simulink model "FIXEDPOINT_SECOND_ORDER_SIGMADELTA_QUANTIZED"  (R2021b)
settings: Solver=VariableStepAuto  StartTime=0.0  StopTime=0.01  MaxStep=1e-8  RelTol=1e-3
libraries: fl_lib x9, nesl_utility x4, dspmlti4 x1
settings Model: FPTShortcutValueString='{{},{''BaselineRun'',1,1,1,''BaselineRun'','''',{},''M'','''',''''},{''EmbeddedRun'',1,1,1,''EmbeddedRun'','''',{},''M'','''',''''}}'  Creator=caccolillo  LastModifiedBy=caccolillo
settings OptimizationCC: BlockReduction=off  ConditionallyExecuteInputs=off
settings DebuggingCC: SignalRangeChecking=warning

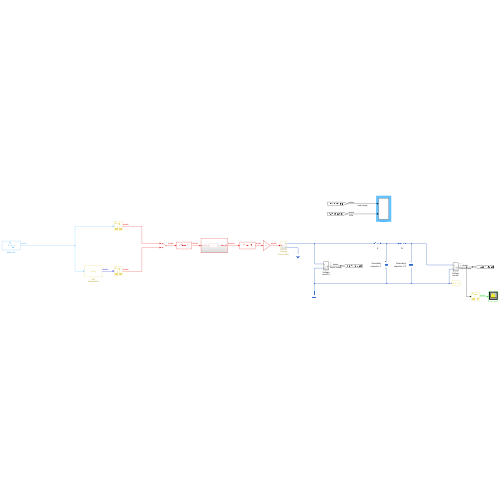
[thumbnail: Simulink's stored preview of the top-level diagram]
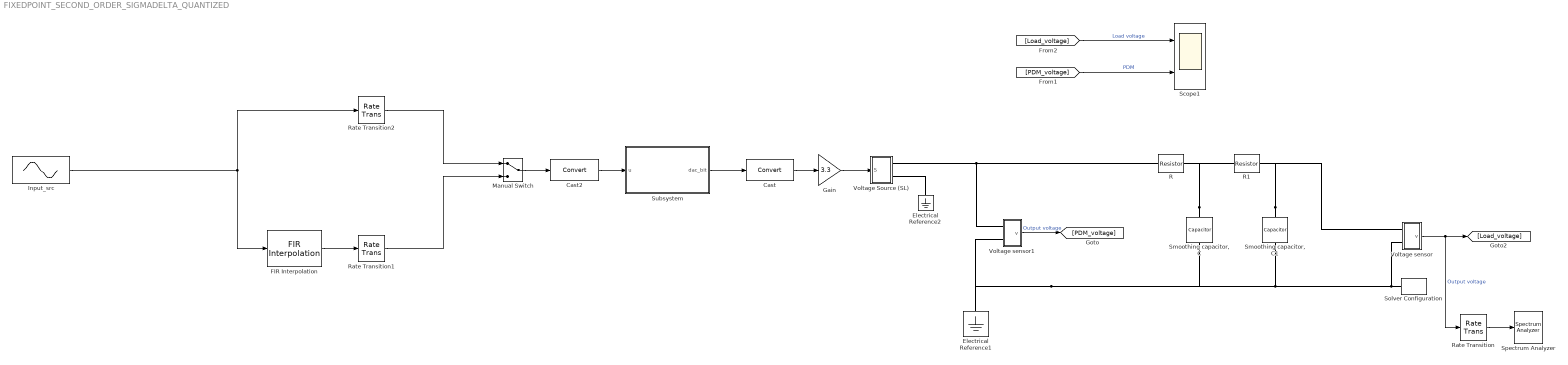
== system FIXEDPOINT_SECOND_ORDER_SIGMADELTA_QUANTIZED ==
  Cast : DataTypeConversion
  Cast2 : DataTypeConversion
  Electrical Reference1 : fl_lib/Electrical/Electrical Elements/Electrical Reference
  Electrical Reference2 : fl_lib/Electrical/Electrical Elements/Electrical Reference
  FIR Interpolation : dspmlti4/FIR Interpolation  FilterSource=Dialog parameters  PrivateCoeffs=0  h=[0.25 0.5 0.75 1.0 0.75 0.5 0.25]  L=4  FilterObject=FINTERP  framing=Allow multirate processing  outputBufInitCond=0  roundingMode=Floor  overflowMode=off  firstCoeffDataTypeStr=Inherit: Same word length as input  firstCoeffMin=[]  firstCoeffMax=[]  firstCoeffLastDataTypeStr=Inherit: Same word length as input  outputDataTypeStr=Inherit: Same as accumulator  outputMin=[]  outputMax=[]  outputLastDataTypeStr=Inherit: Same as accumulator
  Gain : Gain  Gain=3.3
  Input_src : Sin  Amplitude="32  %2^(13-1)"  Frequency=2*pi*440  SampleTime=1/8000
  Manual Switch : ManualSwitch
  R : fl_lib/Electrical/Electrical Elements/Resistor  R=1 kOhm  i_specify=off  i_priority=High  i=0 A  i_nominal_specify=off  i_nominal_unit=A  i_nominal_value=1  v_specify=off  v_priority=High  v=0 V  v_nominal_specify=off  v_nominal_unit=V  v_nominal_value=1
  R1 : fl_lib/Electrical/Electrical Elements/Resistor  R=1 kOhm  i_specify=off  i_priority=High  i=0 A  i_nominal_specify=off  i_nominal_unit=A  i_nominal_value=1  v_specify=off  v_priority=High  v=0 V  v_nominal_specify=off  v_nominal_unit=V  v_nominal_value=1
  Rate Transition : RateTransition  Deterministic=off  OutPortSampleTime=1/100e3
  Rate Transition1 : RateTransition  Deterministic=off  OutPortSampleTime=1/5000000
  Rate Transition2 : RateTransition  Deterministic=off  OutPortSampleTime=1/5000000
  Scope1 : Scope  NumInputPorts=2
  "Smoothing capacitor, C" : fl_lib/Electrical/Electrical Elements/Capacitor  c=10 nF  r=0 Ohm  g=0 1/Ohm  i_specify=off  i_priority=High  i=0 A  i_nominal_specify=off  i_nominal_unit=A  i_nominal_value=1  v_specify=off  v_priority=High  v=0 V  v_nominal_specify=off  v_nominal_unit=V  v_nominal_value=1  vc_specify=on  vc_priority=High  vc=0 V  vc_nominal_specify=off  vc_nominal_unit=V  vc_nominal_value=1
  "Smoothing capacitor, C1" : fl_lib/Electrical/Electrical Elements/Capacitor  c=10 nF  r=0 Ohm  g=0 1/Ohm  i_specify=off  i_priority=High  i=0 A  i_nominal_specify=off  i_nominal_unit=A  i_nominal_value=1  v_specify=off  v_priority=High  v=0 V  v_nominal_specify=off  v_nominal_unit=V  v_nominal_value=1  vc_specify=on  vc_priority=High  vc=0 V  vc_nominal_specify=off  vc_nominal_unit=V  vc_nominal_value=1
  Solver Configuration : nesl_utility/Solver Configuration  PhysicalDomain=network_engine_domain  SubClassName=solver  LeftPortType=input  RightPortType=generic  Tones=[]  Harmonics=[]  SimulateNoise=off  Profile=off  UseLocalSampling=off  EnableSwitchedLinearOptims=on  FrequencyDomain=off  UseCCode=off  RelTol=0.001  AbsTol=1e-06  MinStep=1e-09  ToWorkspace=off  RevertToSquareIcSolve=off  NumHomotopyIterations=100  PhasorMode=off  PhasorModeNumHarmonics=1  DoDC=off  ResidualTolerance=1e-9  UseLocalSolver=off  LocalSolverChoice=NE_BACKWARD_EULER_ADVANCER  LocalSolverSampleTime=1e-7  DoFixedCost=off  MaxNonlinIter=12  MaxModeIter=2  ComputeImpulses=off  ImpulseIterations=2  LinearAlgebra=Sparse  EquationFormulation=NE_TIME_EF  DelaysMemoryBudget=1024  AutomaticFiltering=on  FilteringTimeConstant=0.001  PartitionStorageMethod=AS_NEEDED  PartitionMemoryBudget=1024  PartitionMethod=FAST
      settings: SourceProductBaseCode=PW,SS
  Spectrum Analyzer : SpectrumAnalyzer
  Subsystem : Subsystem
  Voltage Source (SL) : Subsystem
      settings: CopyFcn=set_param(gcb,'LinkStatus','none')
  Voltage sensor : Subsystem
      settings: CopyFcn=set_param(gcb,'LinkStatus','none')
  Voltage sensor1 : Subsystem
      settings: CopyFcn=set_param(gcb,'LinkStatus','none')
  wires:
  [PDM_voltage] -> Scope1/2  "PDM"
  Rate Transition/1 -> Spectrum Analyzer/1
  Voltage sensor/1(v) -> Rate Transition/1, [Load_voltage]  "Output voltage"
  Voltage sensor1/1(v) -> [PDM_voltage]  "Output voltage"
  Gain/1 -> Voltage Source (SL)/1(S)
  [Load_voltage] -> Scope1/1  "Load voltage"
  Cast/1 -> Gain/1
  Input_src/1 -> FIR Interpolation/1, Rate Transition2/1
  FIR Interpolation/1 -> Rate Transition1/1
  Manual Switch/1 -> Cast2/1
  Rate Transition2/1 -> Manual Switch/1
  Rate Transition1/1 -> Manual Switch/2
  Cast2/1 -> Subsystem/1(u)
  Subsystem/1(dac_bit) -> Cast/1
  connections:
  Solver Configuration/RConn1 -- Voltage sensor1/LConn2 -- Electrical Reference1/LConn1 -- "Smoothing capacitor, C"/RConn1 -- "Smoothing capacitor, C1"/RConn1 -- Voltage sensor/LConn2
  "Smoothing capacitor, C"/LConn1 -- R/LConn1 -- R1/RConn1
  "Smoothing capacitor, C1"/LConn1 -- R1/LConn1 -- Voltage sensor/LConn1
  Voltage sensor1/LConn1 -- R/RConn1 -- Voltage Source (SL)/RConn1
  Voltage Source (SL)/RConn2 -- Electrical Reference2/LConn1

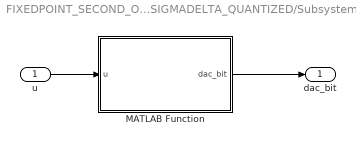
== system FIXEDPOINT_SECOND_ORDER_SIGMADELTA_QUANTIZED/Subsystem ==
  u : Inport
  MATLAB Function : MATLAB Function  TreatAsAtomicUnit=on
  dac_bit : Outport
  wires:
  u/1 -> MATLAB Function/1(u)
  MATLAB Function/1(dac_bit) -> dac_bit/1

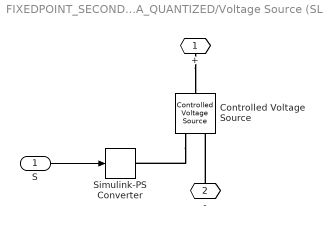
== system FIXEDPOINT_SECOND_ORDER_SIGMADELTA_QUANTIZED/Voltage Source (SL) ==
  S : Inport
  Controlled Voltage Source : fl_lib/Electrical/Electrical Sources/Controlled Voltage Source
  Simulink-PS Converter : nesl_utility/Simulink-PS Converter  PhysicalDomain=network_engine_domain  SubClassName=ps_input  LeftPortType=input  RightPortType=output  PseudoPeriodic=off  Frequencies=[]  NoiseDistribution=none  NoiseParameters=[]  Unit=V  AffineConversion=off  FilteringAndDerivatives=zero  SimscapeFilterOrder=1  InputFilterTimeConstant=.001  UdotUserProvided=0
      settings: SourceProductBaseCode=PW,SS
  + : PMIOPort  Side=Right
  - : PMIOPort  Port=2  Side=Right
  wires:
  S/1 -> Simulink-PS Converter/1
  connections:
  +/RConn1 -- Controlled Voltage Source/LConn1
  -/RConn1 -- Controlled Voltage Source/RConn2
  Controlled Voltage Source/RConn1 -- Simulink-PS Converter/RConn1

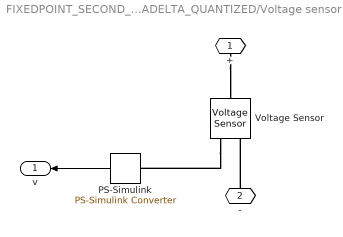
== system FIXEDPOINT_SECOND_ORDER_SIGMADELTA_QUANTIZED/Voltage sensor ==
  PS-Simulink : nesl_utility/PS-Simulink Converter  PhysicalDomain=network_engine_domain  SubClassName=ps_output  LeftPortType=input  RightPortType=output  PseudoPeriodic=off  Frequencies=[]  Unit=V  AffineConversion=off
      settings: SourceProductBaseCode=PW,SS
  Voltage Sensor : fl_lib/Electrical/Electrical Sensors/Voltage Sensor
  + : PMIOPort  Side=Left
  - : PMIOPort  Port=2  Side=Left
  v : Outport
  wires:
  PS-Simulink/1 -> v/1
  connections:
  Voltage Sensor/RConn1 -- PS-Simulink/LConn1
  +/RConn1 -- Voltage Sensor/LConn1
  -/RConn1 -- Voltage Sensor/RConn2

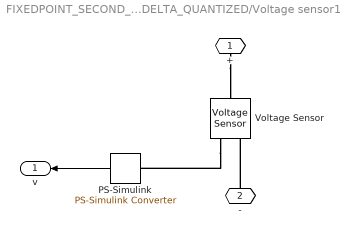
== system FIXEDPOINT_SECOND_ORDER_SIGMADELTA_QUANTIZED/Voltage sensor1 ==
  PS-Simulink : nesl_utility/PS-Simulink Converter  PhysicalDomain=network_engine_domain  SubClassName=ps_output  LeftPortType=input  RightPortType=output  PseudoPeriodic=off  Frequencies=[]  Unit=V  AffineConversion=off
      settings: SourceProductBaseCode=PW,SS
  Voltage Sensor : fl_lib/Electrical/Electrical Sensors/Voltage Sensor
  + : PMIOPort  Side=Left
  - : PMIOPort  Port=2  Side=Left
  v : Outport
  wires:
  PS-Simulink/1 -> v/1
  connections:
  Voltage Sensor/RConn1 -- PS-Simulink/LConn1
  +/RConn1 -- Voltage Sensor/LConn1
  -/RConn1 -- Voltage Sensor/RConn2

== matlab function FIXEDPOINT_SECOND_ORDER_SIGMADELTA_QUANTIZED/Subsystem/MATLAB Function ==
  data: u input; dac_bit output
%auto-generated
function dac_bit = SDM_fcn_fp_fixpt(u)  %#codegen

%% 2nd-order CIFB SDM — double-precision floating-point version
%% u is the audio sample input — same scale as the integer version:
%%   range -4096 to +4095 (13-bit signed full scale)
%%
%% All internal arithmetic uses double precision.
%% Coefficients are the same Q16 integer values divided by 2^16
%% so they represent the same real-valued coefficients as the
%% Verilog/integer implementation.
%%
%% Output: boolean dac_bit (1-bit PDM)

fm = get_fimath();
u = fi(u, 1, 16, 2, fm);

dac_bit = false;

persistent int1 int2
if isempty(int1)
    int1 = fi(0.0, 1, 16, 12, fm);
    int2 = fi(0.0, 1, 16, 11, fm);
end

%% ---------------------------------------------------------------
%  COEFFICIENTS — exact same values as integer version
%  Original integers were Q16 (scaled by 2^16 = 65536)
%  Dividing by 65536 recovers the real-valued coefficient
% ---------------------------------------------------------------
B1 = fi(51138 / 65536, 0, 16, 16, fm);     %  ≈ 0.7803
A1 = fi(51138 / 65536, 0, 16, 16, fm);     %  ≈ 0.7803
C1 =  fi(3493 / 65536, 0, 16, 20, fm);     %  ≈ 0.0533
A2 =  fi(9765 / 65536, 0, 16, 18, fm);     %  ≈ 0.1490

%% ---------------------------------------------------------------
%  INPUT NORMALISATION
%  Map the 13-bit signed integer input to the [-1, +1] range
%  expected by the normalised SDM coefficients above.
%
%  +4095 → +0.9998
%  -4096 → -1.0
% ---------------------------------------------------------------
u_d = fi(double(u), 1, 16, 2, fm);

%% Clamp to 13-bit signed range
if u_d >  fi(4095, 0, 12, 0, fm), u_d(:) =  4095; end
if u_d < fi(-4096, 1, 13, 0, fm), u_d(:) = -4096; end

%% Normalise to [-1, +1]
u_norm = fi(fi_div_by_shift(u_d, 12), 1, 16, 14, fm);

%% ---------------------------------------------------------------
%  QUANTIZER — sign of int2
% ---------------------------------------------------------------
if int2 >= fi(0.0, 0, 1, 0, fm)
    dac_bit(:) = true;
    dac_val = fi(+1.0, 1, 16, 14, fm);
else
    dac_bit(:) = false;
    dac_val = fi(-1.0, 1, 16, 14, fm);
end

%% ---------------------------------------------------------------
%  INTEGRATOR 1: int1[n] = B1*u_norm[n] + int1[n-1] - A1*dac_val
% ---------------------------------------------------------------
int1(:) = fi_signed(int1 + B1 * u_norm) - A1 * dac_val;

%% Saturation — match integer version's ±524288/65536 = ±8.0 range
if int1 >  fi(8.0, 0, 4, 0, fm), int1(:) =  8.0; end
if int1 < fi(-8.0, 1, 4, 0, fm), int1(:) = -8.0; end

%% ---------------------------------------------------------------
%  INTEGRATOR 2: int2[n] = C1*int1[n] + int2[n-1] - A2*dac_val
% ---------------------------------------------------------------
int2(:) = fi_signed(int2 + C1 * int1) - A2 * dac_val;

%% Saturation
if int2 >  fi(8.0, 0, 4, 0, fm), int2(:) =  8.0; end
if int2 < fi(-8.0, 1, 4, 0, fm), int2(:) = -8.0; end

end



function y = fi_div_by_shift(a,shift_len)
    coder.inline( 'always' );
    if isfi( a )
        nt = numerictype( a );
        fm = fimath( a );
        nt_bs = numerictype( nt.Signed, nt.WordLength + shift_len, nt.FractionLength + shift_len );
        y = bitsra( fi( a, nt_bs, fm ), shift_len );
    else
        y = a / 2 ^ shift_len;
    end
end


function y = fi_signed(a)
    coder.inline( 'always' );
    if isfi( a ) && ~(issigned( a ))
        nt = numerictype( a );
        new_nt = numerictype( 1, nt.WordLength + 1, nt.FractionLength );
        y = fi( a, new_nt, fimath( a ) );
    else
        y = a;
    end
end

function fm = get_fimath()
	fm = fimath('RoundingMethod', 'Floor',...
	     'OverflowAction', 'Wrap',...
	     'ProductMode','FullPrecision',...
	     'MaxProductWordLength', 128,...
	     'SumMode','FullPrecision',...
	     'MaxSumWordLength', 128);
end
